simulink model "mdaqdemo_urecv"  (R2014b)
settings: Solver=FixedStepDiscrete  SolverMode=SingleTasking  StartTime=0.0  StopTime=inf  FixedStep=0.1  RelTol=1e-3
libraries: etargetslib x1
settings Model: SimulationMode=external  Creator=peselnikmg  LastModifiedBy=peselnikmg
settings OptimizationCC: OptimizeModelRefInitCode=on  LifeSpan=1
settings DebuggingCC: UnderspecifiedInitializationDetection=Classic  MergeDetectMultiDrivingBlocksExec=none
settings HardwareCC: ProdBitPerLong=40  ProdLargestAtomicInteger=Integer  ProdIntDivRoundTo=Zero  ProdEndianess=LittleEndian  ProdHWDeviceType=Texas Instruments->C6000
settings RTWCC: SystemTargetFile=microdaq.tlc  TemplateMakefile=microdaq.tmf  PostCodeGenCommand=microdaq_postcodegen(buildInfo)  Description=MicroDAQ Real-Time Measurement System  GenerateReport=on  ProcessScript=microdaq_make_rtw_hook  IncludeHyperlinkInReport=on  LaunchReport=on  GenerateTraceInfo=on  GenerateTraceReport=on  GenerateTraceReportSl=on  GenerateTraceReportSf=on  GenerateTraceReportEml=on
settings CodeAppCC: IgnoreCustomStorageClasses=off
settings STFCustomTargetCC: CodeReplacementLibrary=TI C674x  CombineOutputUpdateFcns=on  ERTCustomFileBanners=on  SupportContinuousTime=off  SupportNonInlinedSFcns=off  MATLABClassNameForMDSCustomization=Simulink.SoftwareTarget.ERTCustomization  GRTInterface=off  SystemTargetFile=microdaq.tlc
settings ERTTargetCC: CodeReplacementLibrary=TI C674x  ParMdlRefBuildCompliant=off  CompOptLevelCompliant=off  ConcurrentExecutionCompliant=off  ERTFirstTimeCompliant=off  ModelStepFunctionPrototypeControlCompliant=off  CPPClassGenCompliant=off  ExtMode=on  ExtModeStaticAlloc=on  ExtModeStaticAllocSize=10485760  ExtModeMexArgs=getpref('microdaq','TargetIP') 1 4344  InlinedParameterPlacement=NonHierarchical  ERTCustomFileTemplate=microdaq_main.tlc

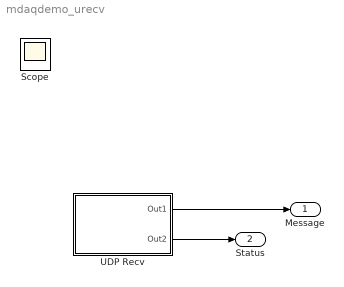
== system mdaqdemo_urecv ==
  UDP Recv : Subsystem  mask(UDP Recv){IPAddrStr='10.10.1.10', Port=5001, Blocking=off, Timeout=250, Datatype=uint8, SizePack=1, SampleTime=-1}
      mask prompts: IPAddrStr "Remote IP address:"; Port "Remote port:"; Timeout "Timeout (ms):"; Datatype "Data type:"; SizePack "Message size (in data type units):"; SampleTime "Sample time:"
      mask help: Receive UDP packets from given IP port and address.
      mask init:
      | % Convert string IP Address to bytes
      | % for use in S-function
      | IPAddr = double(IPAddrStr);
      | % UDP Protocol
      | Protocol = 1;
      | % Construct data type expression for Pack block
      | %packdt = repmat({Datatype},SizePack,1);
      | packdt = {Datatype};
      | % Any better way to find data type size?
      | eval(['dummy = ',Datatype,'(0);']);
      | dummy = whos('dummy');
      | Size = SizePack*dummy.bytes;
      mask TypeOptions Datatype: double | single | uint8 | uint16 | uint32 | int8 | int16 | int32 | boolean
      mask Display:
      | color('blue');
      | text(0.98, 0.13, 'MicroDAQ', 'horizontalalignment', 'right');
      | color('black');
      | fprintf('UDP Recv\n\n\n');
      | color('gray');
  Message : Outport
  Status : Outport  Port=2
  Scope : Scope  NumInputPorts=2
      settings: YMin=-1~-12  YMax=1~-10
  wires:
  UDP Recv/1(Out1) -> Message/1
  UDP Recv/2(Out2) -> Status/1

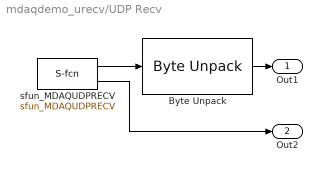
== system mdaqdemo_urecv/UDP Recv ==
  Byte Unpack : etargetslib/Byte Unpack  dimensions={SizePack}  datatypes=packdt  byteAlign=1
  sfun_MDAQUDPRECV : S-Function  FunctionName=sfun_MDAQUDPRECV  Parameters=IPAddr, Port, Blocking, Timeout, Protocol, Size, SampleTime  EnableBusSupport=off
  Out1 : Outport
  Out2 : Outport  Port=2
  wires:
  sfun_MDAQUDPRECV/1 -> Byte Unpack/1
  sfun_MDAQUDPRECV/2 -> Out2/1
  Byte Unpack/1 -> Out1/1
